simulink model "robotAGV"  (R2022a)
settings: Solver=FixedStepAuto  StartTime=0.0  StopTime=inf  FixedStep=0.1  RelTol=1e-3  EnableMultiTasking=on
libraries: mobileRoboticsLib x1
settings Model: PacingRate=0.200000  Creator=emanu  LastModifiedBy=emanu
settings SolverCC: AlgebraicLoopSolver=TrustRegion  AutoInsertRateTranBlk=on
settings DataIOCC: LimitDataPoints=on
settings OptimizationCC: LifeSpan=inf
settings DebuggingCC: UnconnectedInputMsg=warning  UnconnectedOutputMsg=warning  UnconnectedLineMsg=warning  AllowSymbolicDim=off  SFUnexpectedBacktrackingDiag=warning  SFNoUnconditionalDefaultTransitionDiag=warning  SFExecutionAtInitializationDiag=none  ArithmeticOperatorsInVariantConditions=warning
settings SFSimCC: SimUseLocalCustomCode=off  CustomCodeUndefinedFunction=UseInterfaceOnly
settings RTWCC: RTWUseLocalCustomCode=off  DLArmComputeVersion=19.05
settings CodeAppCC: StateflowObjectComments=on
settings GRTTargetCC: TargetLangStandard=C89/C90 (ANSI)
settings ConfigComp: CovMetricSettings=dw  CovSaveCumulativeToWorkspaceVar=on  CovSaveSingleToWorkspaceVar=on  CovExternalEMLEnable=off  CovSFcnEnable=off

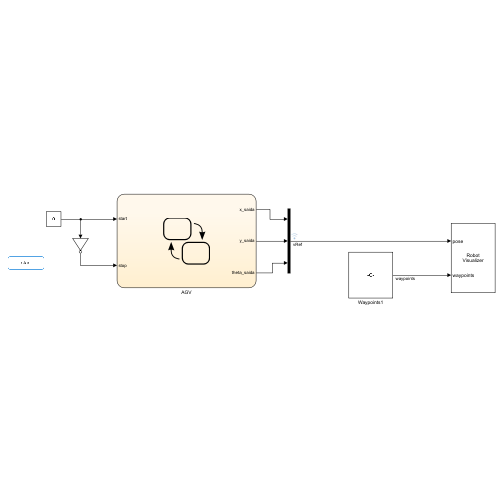
[thumbnail: Simulink's stored preview of the top-level diagram]
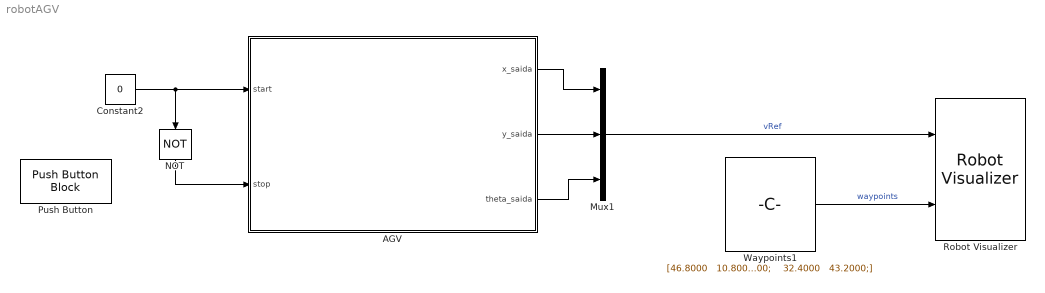
== system robotAGV ==
  AGV : Stateflow chart  TreatAsAtomicUnit=on
  Constant2 : Constant  Value=0
  Mux1 : Mux  Inputs=3
  NOT : Logic  Operator=NOT  IconShape=distinctive  AllPortsSameDT=off  OutDataTypeStr=boolean
  Push Button : PushButtonBlock  ButtonText=start  ButtonType=Latch  OffValue=0.000000
  Robot Visualizer : mobileRoboticsLib/Environments/Robot Visualizer  robotRadius=0.8  showTrajectory=on  hasWaypoints=on  hasLidar=off  sensorOffset=[ 0, 0 ]  scanAngles=[ pi/4, 0, -pi/4 ]  hasObjDetector=off  objDetectorOffset=[ 0, 0 ]  objDetectorAngle=0  objDetectorFOV=pi/4  objDetectorMaxRange=5  objectColors=[ 1, 0, 0; 0, 1, 0; 0, 0, 1 ]  objectMarkers=s
  Waypoints1 : Constant  Value=|
      | [46.8000   10.8000;
      |    45.0000   10.8000;
      |    43.2000   10.8000;
      |    41.4000   10.8000;
      |    39.6000   10.8000;
      |    37.8000   12.6000;
      |    36.0000   12.6000;
      |    34.2000   12.6000;
      |    32.4000   14.4000;
      |    30.6000   14.4000;
      |    30.6000   16.2000;
      |    28.8000   16.2000;
      |    27.0000   18.0000;
      |    25.2000   18.0000;
      |    25.2000   19.8000;
      |    23.4000   19.8000;
      |    21.6000   21.6000;
      |    19.8000   23.4000;
      |    19.8000   25.2000;
      |    18.0000   25.2000;
      |    18.0000   27.0000;
      |    18.0000   28.8000;
      |    18.0000   30.6000;
      |    18.0000   32.4000;
      |    18.0000   34.2000;
      |    18.0000   36.0000;
      |    18.0000   37.8000;
      |    19.8000   37.8000;
      |    21.6000   37.8000;
      |    21.6000   39.6000;
      |    23.4000   39.6000;
      |    25.2000   39.6000;
      |    27.0000   39.6000;
      |    28.8000   41.4000;
      |    30.6000   41.4000;
      |    32.4000   43.2000;
      |    32.4000   45.0000;
      |    34.2000   45.0000;
      |    36.0000   46.8000;
      |    36.0000   48.6000;
      |    36.0000   50.4000;
      |    36.0000   52.2000;
      |    36.0000   54.0000;
      |    36.0000   55.8000;
      |    36.0000   57.6000;
      |    34.2000   57.6000;
      |    34.2000   59.4000;
      |    34.2000   61.2000;
      |    34.2000   63.0000;
      |    34.2000   64.8000;
      |    36.0000   64.8000;
      |    36.0000   66.6000;
      |    37.8000   66.6000;
      |    37.8000   68.4000;
      |    39.6000   68.4000;
      |    39.6000   70.2000;
      |    41.4000   70.2000;
      |    43.2000   72.0000;
      |    45.0000   72.0000;
      |    45.0000   73.8000;
      |    46.8000   73.8000;
      |    48.6000   73.8000;
      |    50.4000   75.6000;
      |    52.2000   75.6000;
      |    54.0000   75.6000;
      |    54.0000   73.8000;
      |    55.8000   73.8000;
      |    57.6000   73.8000;
      |    59.4000   72.0000;
      |    61.2000   70.2000;
      |    63.0000   70.2000;
      |    64.8000   70.2000;
      |    64.8000   68.4000;
      |    66.6000   68.4000;
      |    68.4000   66.6000;
      |    68.4000   64.8000;
      |    68.4000   63.0000;
      |    70.2000   61.2000;
      |    70.2000   59.4000;
      |    68.4000   57.6000;
      |    68.4000   55.8000;
      |    68.4000   54.0000;
      |    68.4000   52.2000;
      |    66.6000   52.2000;
      |    64.8000   50.4000;
      |    63.0000   50.4000;
      |    61.2000   48.6000;
      |    61.2000   48.6000;
      |    59.4000   46.8000;
      |    57.6000   46.8000;
      |    55.8000   45.0000;
      |    54.0000   45.0000;
      |    52.2000   43.2000;
      |    52.2000   41.4000;
      |    50.4000   41.4000;
      |    50.4000   39.6000;
      |    48.6000   39.6000;
      |    48.6000   37.8000;
      |    48.6000   36.0000;
      |    46.8000   34.2000;
      |    46.8000   32.4000;
      |    48.6000   30.6000;
      |    50.4000   28.8000;
      |    52.2000   28.8000;
      |    52.2000   27.0000;
      |    54.0000   27.0000;
      |    55.8000   27.0000;
      |    55.8000   25.2000;
      |    57.6000   25.2000;
      |    59.4000   23.4000;
      |    61.2000   21.6000;
      |    61.2000   19.8000;
      |    61.2000   18.0000;
      |    61.2000   16.2000;
      |    61.2000   14.4000;
      |    59.4000   14.4000;
      |    57.6000   12.6000;
      |    55.8000   12.6000;
      |    54.0000   12.6000;
      |    52.2000   12.6000;
      |    52.2000   10.8000;
      |    50.4000   10.8000;
      |    48.6000   10.8000;
      |    61.2000   70.2000;
      |    68.4000   63.0000;
      |    70.2000   59.4000;
      |    43.2000   10.8000;
      |    32.4000   43.2000;]
  wires:
  AGV/3(theta_saida) -> Mux1/3
  AGV/2(y_saida) -> Mux1/2
  Constant2/1 -> NOT/1, AGV/1(start)
  AGV/1(x_saida) -> Mux1/1
  Mux1/1 -> Robot Visualizer/1  "vRef"
  NOT/1 -> AGV/2(stop)
  Waypoints1/1 -> Robot Visualizer/2  "waypoints"

== stateflow chart robotAGV/AGV ==
  settings: updateMethod=CONTINUOUS
  state STRAIGHT
    du:
    x_dot = a*cos(theta);
    y_dot = a*sin(theta);
    theta_dot = 0;
    x_saida = x;
    y_saida = y;
    theta_saida = theta;
  state RIGHT
    du:
    x_dot = a*cos(theta);
    y_dot = a*sin(theta);
    theta_dot = -pi;
    x_saida = x;
    y_saida = y;
    theta_saida = theta;
  state LEFT
    du:
    x_dot = a*cos(theta);
    y_dot = a*sin(theta);
    theta_dot = pi;
    x_saida = x;
    y_saida = y;
    theta_saida = theta;
  state STOP
    du:
    x_dot = 0;
    y_dot = 0;
    theta_dot = 0;
    x_saida = x;
    y_saida = y;
    theta_saida = theta;
  STRAIGHT -> STRAIGHT [order 4] : [~stop]{idx=idx+1}
  RIGHT -> RIGHT [order 4] : [~stop]{idx=idx+1}
  STRAIGHT -> RIGHT [order 3] : [~stop && fct(x,y,theta,idx) > e2]{idx=idx+1}
  RIGHT -> STRAIGHT [order 1] : [~stop && abs(fct(x,y,theta,idx))< e1]{idx=idx+1}
  STOP -> STRAIGHT : [start  && idx < numPoints ]{idx=idx+1}
  RIGHT -> STOP [order 2] : [stop || idx==numPoints]
  RIGHT -> LEFT [order 3] : [~stop && fct(x,y,theta,idx) < -e2]{idx=idx+1}
  LEFT -> RIGHT [order 2] : [ ~stop && fct(x,y,theta,idx) >  e2]{idx=idx+1}
  STRAIGHT -> STOP [order 1] : [stop || idx==numPoints]
  STRAIGHT -> LEFT [order 2] : [~stop && fct(x,y,theta,idx) < -e2 ]{idx=idx+1}
  LEFT -> STRAIGHT [order 3] : [~stop && abs(fct(x,y,theta,idx))< e1 ]{idx=idx+1}
  LEFT -> LEFT [order 4] : [~stop]{idx=idx+1}
  (default) -> STOP : {x = x0;
      | y = y0;
      | theta = theta0;
      | idx = 2}
  LEFT -> STOP [order 1] : [stop || idx==numPoints]
  data: erro function_output; x1 function_input; y1 function_input; theta1 function_input; ind function_input; x_saida output; y_saida output; y0 local =10.8; x0 local =46.8; theta0 local =pi; start input; stop input; e2 local =0.5; e1 local =0.1; theta_saida output; x local; y local; theta local; a constant double =16; idx local; numPoints local double =128
  data x settings: updateMethod=SF_CONTINUOUS_TIME_DATA
  data y settings: updateMethod=SF_CONTINUOUS_TIME_DATA
  data theta settings: updateMethod=SF_CONTINUOUS_TIME_DATA
  function erro = fct(x1,y1,theta1,ind):
    | function erro = fct(x1,y1,theta1,ind)
    | 
    |         u=[46.8000   10.8000;
    |            45.0000   10.8000;
    |            43.2000   10.8000;
    |            41.4000   10.8000;
    |            39.6000   10.8000;
    |            37.8000   12.6000;
    |            36.0000   12.6000;
    |            34.2000   12.6000;
    |            32.4000   14.4000;
    |            30.6000   14.4000;
    |            30.6000   16.2000;
    |            28.8000   16.2000;
    |            27.0000   18.0000;
    |            25.2000   18.0000;
    |            25.2000   19.8000;
    |            23.4000   19.8000;
    |            21.6000   21.6000;
    |            19.8000   23.4000;
    |            19.8000   25.2000;
    |            18.0000   25.2000;
    |            18.0000   27.0000;
    |            18.0000   28.8000;
    |            18.0000   30.6000;
    |            18.0000   32.4000;
    |            18.0000   34.2000;
    |            18.0000   36.0000;
    |            18.0000   37.8000;
    |            19.8000   37.8000;
    |            21.6000   37.8000;
    |            21.6000   39.6000;
    |            23.4000   39.6000;
    |            25.2000   39.6000;
    |            27.0000   39.6000;
    |            28.8000   41.4000;
    |            30.6000   41.4000;
    |            32.4000   43.2000;
    |            32.4000   45.0000;
    |            34.2000   45.0000;
    |            36.0000   46.8000;
    |            36.0000   48.6000;
    |            36.0000   50.4000;
    |            36.0000   52.2000;
    |            36.0000   54.0000;
    |            36.0000   55.8000;
    |            36.0000   57.6000;
    |            34.2000   57.6000;
    |            34.2000   59.4000;
    |            34.2000   61.2000;
    |            34.2000   63.0000;
    |            34.2000   64.8000;
    |            36.0000   64.8000;
    |            36.0000   66.6000;
    |            37.8000   66.6000;
    |            37.8000   68.4000;
    |            39.6000   68.4000;
    |            39.6000   70.2000;
    |            41.4000   70.2000;
    |            43.2000   72.0000;
    |            45.0000   72.0000;
    |            45.0000   73.8000;
    |            46.8000   73.8000;
    |            48.6000   73.8000;
    |            50.4000   75.6000;
    |            52.2000   75.6000;
    |            54.0000   75.6000;
    |            54.0000   73.8000;
    |            55.8000   73.8000;
    |            57.6000   73.8000;
    |            59.4000   72.0000;
    |            61.2000   70.2000;
    |            63.0000   70.2000;
    |            64.8000   70.2000;
    |            64.8000   68.4000;
    |            66.6000   68.4000;
    |            68.4000   66.6000;
    |            68.4000   64.8000;
    |            68.4000   63.0000;
    |            70.2000   61.2000;
    |            70.2000   59.4000;
    |            68.4000   57.6000;
    |            68.4000   55.8000;
    |            68.4000   54.0000;
    |            68.4000   52.2000;
    |            66.6000   52.2000;
    |            64.8000   50.4000;
    |            63.0000   50.4000;
    |            61.2000   48.6000;
    |            61.2000   48.6000;
    |            59.4000   46.8000;
    |            57.6000   46.8000;
    |            55.8000   45.0000;
    |            54.0000   45.0000;
    |            52.2000   43.2000;
    |            52.2000   41.4000;
    |            50.4000   41.4000;
    |            50.4000   39.6000;
    |            48.6000   39.6000;
    |            48.6000   37.8000;
    |            48.6000   36.0000;
    |            46.8000   34.2000;
    |            46.8000   32.4000;
    |            48.6000   30.6000;
    |            50.4000   28.8000;
    |            52.2000   28.8000;
    |            52.2000   27.0000;
    |            54.0000   27.0000;
    |            55.8000   27.0000;
    |            55.8000   25.2000;
    |            57.6000   25.2000;
    |            59.4000   23.4000;
    |            61.2000   21.6000;
    |            61.2000   19.8000;
    |            61.2000   18.0000;
    |            61.2000   16.2000;
    |            61.2000   14.4000;
    |            59.4000   14.4000;
    |            57.6000   12.6000;
    |            55.8000   12.6000;
    |            54.0000   12.6000;
    |            52.2000   12.6000;
    |            52.2000   10.8000;
    |            50.4000   10.8000;
    |            48.6000   10.8000;
    |            61.2000   70.2000;
    |            68.4000   63.0000;
    |            70.2000   59.4000;
    |            43.2000   10.8000;
    |            32.4000   43.2000;];
    | 
    |     pose1 = u(ind,1) - x1 ;
    |     pose2 = u(ind,2) - y1 ; 
    |     ang = angdiff(theta1,atan2(pose2,pose1));
    |   
    |     if (ang < 0)
    |            d = sqrt(pose1^2 + pose2^2);
    |     else
    |            d = -sqrt(pose1^2 + pose2^2);
    |     end
    |     erro = d;
